simulink model "bilat_teleop_multiDOF"  (R2017a)
settings: Solver=VariableStepAuto  StartTime=0.0  StopTime=10.0  RelTol=1e-3
values from neighbouring files (symbols this model uses):
  Am = [1 0; 0 1]    [bilat_teleop_multiDOF_params.m]
  As = [1 0; 0 1]    [bilat_teleop_multiDOF_params.m]
  Be = [0 0; 0 0]    [bilat_teleop_multiDOF_params.m]    (also in sampled_data_bilat_teleop_tavakoli_params.m = 0; sampled_data_bilat_teleop_time_delay_params.m = 0)
  Bh = [0 0; 0 0]    [bilat_teleop_multiDOF_params.m]    (also in sampled_data_bilat_teleop_tavakoli_params.m = 0.1; sampled_data_bilat_teleop_time_delay_params.m = 0.1)
  Bm = [1 0; 0 1]    [bilat_teleop_multiDOF_params.m]    (also in bilat_teleop_time_delay_params.m = 0; sampled_data_bilat_teleop_tavakoli_params.m = 0.1; sampled_data_bilat_teleop_time_delay_params.m = 0.1)
  Bs = [1 0; 0 1]    [bilat_teleop_multiDOF_params.m]    (also in bilat_teleop_time_delay_params.m = 0; sampled_data_bilat_teleop_tavakoli_params.m = 0.1; sampled_data_bilat_teleop_time_delay_params.m = 0.1)
  Ke = 0.142826110455    [Oct12workspace.mat]    (also in Test_apparatus_simulation.m; bilat_teleop_multiDOF_params.m = [0 0; 0 0]; sampled_data_bilat_teleop_tavakoli_params.m = 0; sampled_data_bilat_teleop_time_delay_params.m = 0)
  Kh = [0 0; 0 0]    [bilat_teleop_multiDOF_params.m]    (also in sampled_data_bilat_teleop_tavakoli_params.m = 0; sampled_data_bilat_teleop_time_delay_params.m = 0)
  Me = [0 0; 0 0]    [bilat_teleop_multiDOF_params.m]    (also in sampled_data_bilat_teleop_tavakoli_params.m = 0; sampled_data_bilat_teleop_time_delay_params.m = 0)
  Mh = [0 0; 0 0]    [bilat_teleop_multiDOF_params.m]    (also in sampled_data_bilat_teleop_tavakoli_params.m = 0.1; sampled_data_bilat_teleop_time_delay_params.m = 0.1)
libraries: simulink x2
settings Model: Creator=salou  LastModifiedBy=salou

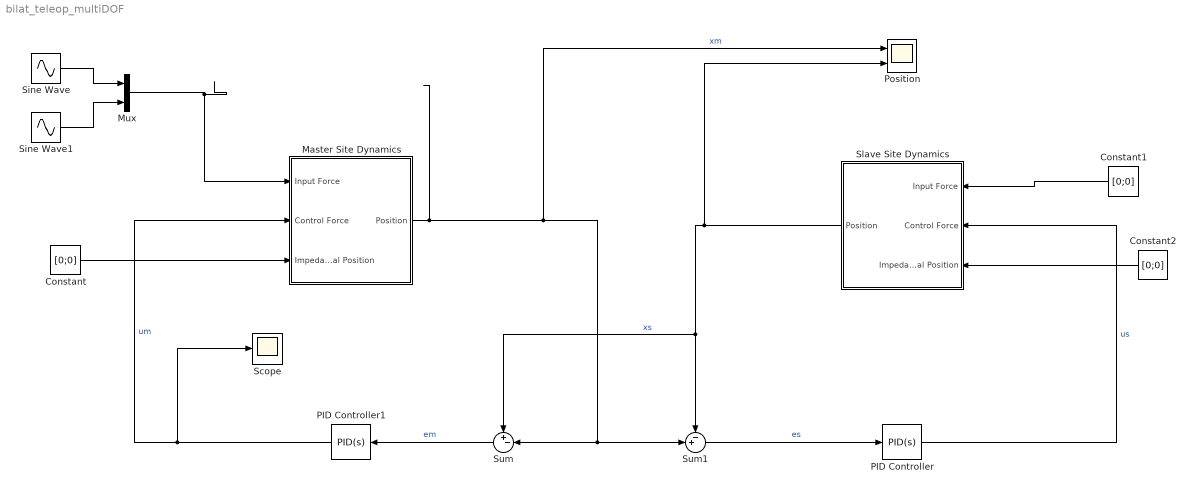
== system bilat_teleop_multiDOF ==
  Constant : Constant  Value=[0;0]
  Constant1 : Constant  Value=[0;0]
  Constant2 : Constant  Value=[0;0]
  Master Site Dynamics : Subsystem
  Mux : Mux  Inputs=2
  PID Controller : simulink/Continuous/PID Controller  Controller=PID  TimeDomain=Continuous-time  SampleTime=-1  IntegratorMethod=Forward Euler  FilterMethod=Forward Euler  Form=Parallel  UseFilter=on  ControllerParametersSource=internal  P=[1 1]  I=[0 0]  D=[0 0]  N=100  InitialConditionSource=internal  InitialConditionForIntegrator=0  InitialConditionForFilter=0  ExternalReset=none  LimitOutput=off  UpperSaturationLimit=inf  LowerSaturationLimit=-inf  LinearizeAsGain=on  AntiWindupMode=none  Kb=1  TrackingMode=off  Kt=1  PParamMin=[]  PParamMax=[]  IParamMin=[]  IParamMax=[]  DParamMin=[]  DParamMax=[]  NParamMin=[]  NParamMax=[]  KbParamMin=[]  KbParamMax=[]  KtParamMin=[]  KtParamMax=[]  POutMin=[]  POutMax=[]  IOutMin=[]  IOutMax=[]  DOutMin=[]  DOutMax=[]  NOutMin=[]  NOutMax=[]  KbOutMin=[]  KbOutMax=[]  KtOutMin=[]  KtOutMax=[]  IntegratorOutMin=[]  IntegratorOutMax=[]  FilterOutMin=[]  FilterOutMax=[]  SumOutMin=[]  SumOutMax=[]  SumI1OutMin=[]  SumI1OutMax=[]  SumI2OutMin=[]  SumI2OutMax=[]  SumI3OutMin=[]  SumI3OutMax=[]  SumDOutMin=[]  SumDOutMax=[]  SaturationOutMin=[]  SaturationOutMax=[]  IntegratorContinuousStateAttributes=''  IntegratorStateMustResolveToSignalObject=off  IntegratorRTWStateStorageClass=Auto  FilterContinuousStateAttributes=''  FilterStateMustResolveToSignalObject=off  FilterRTWStateStorageClass=Auto  DifferentiatorICPrevScaledInput=0  DifferentiatorOutMin=[]  DifferentiatorOutMax=[]  InitialConditionSetting=State (most efficient)
  PID Controller1 : simulink/Continuous/PID Controller  Controller=PID  TimeDomain=Continuous-time  SampleTime=-1  IntegratorMethod=Forward Euler  FilterMethod=Forward Euler  Form=Parallel  UseFilter=on  ControllerParametersSource=internal  P=[1 1]  I=[0 0]  D=[0 0]  N=100  InitialConditionSource=internal  InitialConditionForIntegrator=0  InitialConditionForFilter=0  ExternalReset=none  LimitOutput=off  UpperSaturationLimit=inf  LowerSaturationLimit=-inf  LinearizeAsGain=on  AntiWindupMode=none  Kb=1  TrackingMode=off  Kt=1  PParamMin=[]  PParamMax=[]  IParamMin=[]  IParamMax=[]  DParamMin=[]  DParamMax=[]  NParamMin=[]  NParamMax=[]  KbParamMin=[]  KbParamMax=[]  KtParamMin=[]  KtParamMax=[]  POutMin=[]  POutMax=[]  IOutMin=[]  IOutMax=[]  DOutMin=[]  DOutMax=[]  NOutMin=[]  NOutMax=[]  KbOutMin=[]  KbOutMax=[]  KtOutMin=[]  KtOutMax=[]  IntegratorOutMin=[]  IntegratorOutMax=[]  FilterOutMin=[]  FilterOutMax=[]  SumOutMin=[]  SumOutMax=[]  SumI1OutMin=[]  SumI1OutMax=[]  SumI2OutMin=[]  SumI2OutMax=[]  SumI3OutMin=[]  SumI3OutMax=[]  SumDOutMin=[]  SumDOutMax=[]  SaturationOutMin=[]  SaturationOutMax=[]  IntegratorContinuousStateAttributes=''  IntegratorStateMustResolveToSignalObject=off  IntegratorRTWStateStorageClass=Auto  FilterContinuousStateAttributes=''  FilterStateMustResolveToSignalObject=off  FilterRTWStateStorageClass=Auto  DifferentiatorICPrevScaledInput=0  DifferentiatorOutMin=[]  DifferentiatorOutMax=[]  InitialConditionSetting=State (most efficient)
  Position : Scope  NumInputPorts=2
  Scope : Scope
  Sine Wave : Sin  SampleTime=0
  Sine Wave1 : Sin  Amplitude=2  SampleTime=0
  Slave Site Dynamics : Subsystem
  Sum : Sum  Inputs=+-|
  Sum1 : Sum  Inputs=-+|
  wires:
  Mux/1 -> Master Site Dynamics/1(Input Force)
  PID Controller1/1 -> Scope/1, Master Site Dynamics/2(Control Force)  "um"
  Constant/1 -> Master Site Dynamics/3(Impedance Virtual Position)
  Master Site Dynamics/1(Position) -> Position/1, Sum/2, Sum1/2  "xm"
  Constant1/1 -> Slave Site Dynamics/1(Input Force)
  Slave Site Dynamics/1(Position) -> Position/2, Sum/1, Sum1/1  "xs"
  Constant2/1 -> Slave Site Dynamics/3(Impedance Virtual Position)
  PID Controller/1 -> Slave Site Dynamics/2(Control Force)  "us"
  Sum/1 -> PID Controller1/1  "em"
  Sum1/1 -> PID Controller/1  "es"
  Sine Wave/1 -> Mux/1
  Sine Wave1/1 -> Mux/2

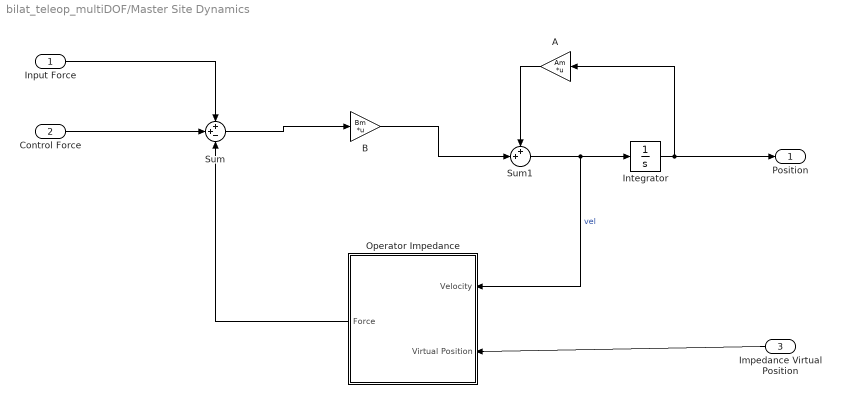
== system bilat_teleop_multiDOF/Master Site Dynamics ==
  Input Force : Inport
  Control Force : Inport  Port=2
  Impedance Virtual Position : Inport  Port=3
  A : Gain  Gain=Am  Multiplication=Matrix(K*u)
  B : Gain  Gain=Bm  Multiplication=Matrix(K*u)
  Integrator : Integrator
  Operator Impedance : Subsystem
  Sum : Sum  Inputs=++-
  Sum1 : Sum  Inputs=++|
  Position : Outport
  wires:
  Input Force/1 -> Sum/1
  Sum1/1 -> Integrator/1, Operator Impedance/1(Velocity)  "vel"
  A/1 -> Sum1/1
  Impedance Virtual Position/1 -> Operator Impedance/2(Virtual Position)
  Operator Impedance/1(Force) -> Sum/3
  B/1 -> Sum1/2
  Sum/1 -> B/1
  Integrator/1 -> Position/1, A/1
  Control Force/1 -> Sum/2

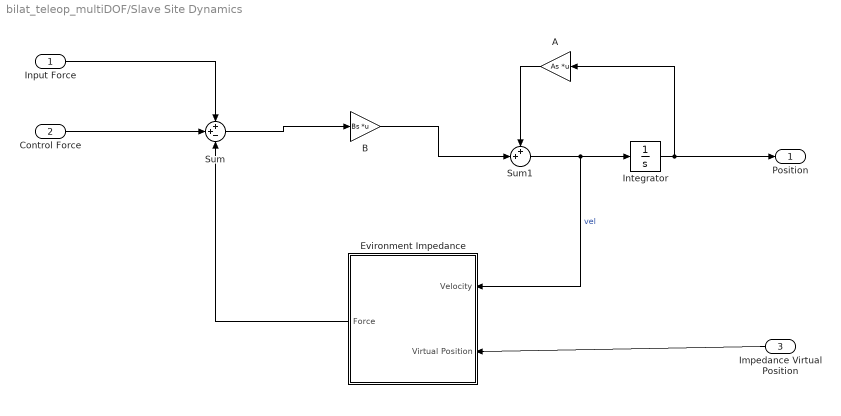
== system bilat_teleop_multiDOF/Slave Site Dynamics ==
  Input Force : Inport
  Control Force : Inport  Port=2
  Impedance Virtual Position : Inport  Port=3
  A : Gain  Gain=As  Multiplication=Matrix(K*u)
  B : Gain  Gain=Bs  Multiplication=Matrix(K*u)
  Evironment Impedance : Subsystem
  Integrator : Integrator
  Sum : Sum  Inputs=++-
  Sum1 : Sum  Inputs=++|
  Position : Outport
  wires:
  Input Force/1 -> Sum/1
  Sum1/1 -> Integrator/1, Evironment Impedance/1(Velocity)  "vel"
  A/1 -> Sum1/1
  Impedance Virtual Position/1 -> Evironment Impedance/2(Virtual Position)
  Evironment Impedance/1(Force) -> Sum/3
  B/1 -> Sum1/2
  Sum/1 -> B/1
  Integrator/1 -> Position/1, A/1
  Control Force/1 -> Sum/2

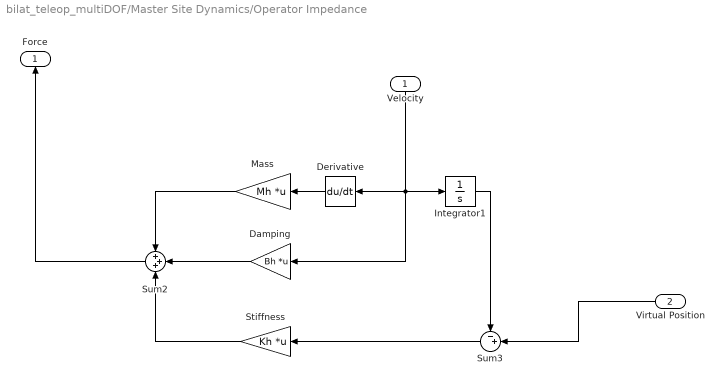
== system bilat_teleop_multiDOF/Master Site Dynamics/Operator Impedance ==
  Velocity : Inport
  Virtual Position : Inport  Port=2
  Damping : Gain  Gain=Bh  Multiplication=Matrix(K*u)
  Derivative : Derivative
  Integrator1 : Integrator
  Mass : Gain  Gain=Mh  Multiplication=Matrix(K*u)
  Stiffness : Gain  Gain=Kh  Multiplication=Matrix(K*u)
  Sum2 : Sum  Inputs=+++
  Sum3 : Sum  Inputs=-+|
  Force : Outport
  wires:
  Integrator1/1 -> Sum3/1
  Derivative/1 -> Mass/1
  Velocity/1 -> Integrator1/1, Damping/1, Derivative/1
  Virtual Position/1 -> Sum3/2
  Sum3/1 -> Stiffness/1
  Damping/1 -> Sum2/2
  Stiffness/1 -> Sum2/3
  Mass/1 -> Sum2/1
  Sum2/1 -> Force/1

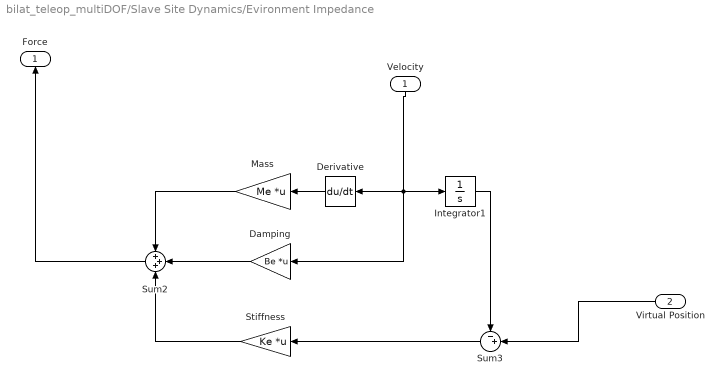
== system bilat_teleop_multiDOF/Slave Site Dynamics/Evironment Impedance ==
  Velocity : Inport
  Virtual Position : Inport  Port=2
  Damping : Gain  Gain=Be  Multiplication=Matrix(K*u)
  Derivative : Derivative
  Integrator1 : Integrator
  Mass : Gain  Gain=Me  Multiplication=Matrix(K*u)
  Stiffness : Gain  Gain=Ke  Multiplication=Matrix(K*u)
  Sum2 : Sum  Inputs=+++
  Sum3 : Sum  Inputs=-+|
  Force : Outport
  wires:
  Integrator1/1 -> Sum3/1
  Derivative/1 -> Mass/1
  Velocity/1 -> Integrator1/1, Damping/1, Derivative/1
  Virtual Position/1 -> Sum3/2
  Sum3/1 -> Stiffness/1
  Damping/1 -> Sum2/2
  Stiffness/1 -> Sum2/3
  Mass/1 -> Sum2/1
  Sum2/1 -> Force/1
